simulink model "sim_test"  (R2021a)
settings: Solver=VariableStepAuto  StartTime=0.0  StopTime=240  RelTol=1e-3
libraries: dspvision x1
settings Model: SimulationMode=accelerator  Creator=Rafid  LastModifiedBy=Rafid

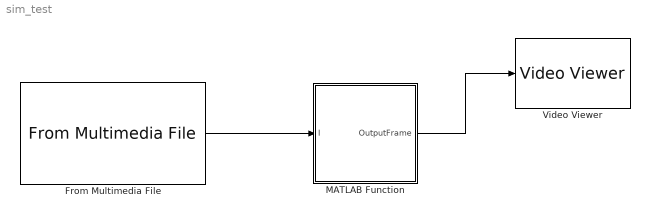
== system sim_test ==
  From Multimedia File : dspvision/From Multimedia File  inputFilename=C:\Users\Rafid\Documents\capstone\DroneCapture2.mp4  readRange=[1 Inf]  loop=on  numPlays=inf  outputStreams=Video only  videoDataType=single  audioDataType=int16  inheritSampleTime=on  userDefinedSampleTime=1/30  noAudioOutput=off  isIntensityVideo=off  fourcc=RGB  colorVideoFormat=One multidimensional signal  outputEOF=off  dataOrg=Column-major  audioFrameSize=1024  computeAudioFrameSize=off  outSamplingMode=Sample based
  MATLAB Function : MATLAB Function  TreatAsAtomicUnit=on
  Video Viewer : VideoViewer  FigPos=[-1919 1461.33333333333 1920 952.666666666667]
  wires:
  MATLAB Function/1(OutputFrame) -> Video Viewer/1
  From Multimedia File/1 -> MATLAB Function/1(I)

== matlab function sim_test/MATLAB Function ==
  data: I input; OutputFrame output
function OutputFrame = fcn(I)
    OutputFrame = ones(size(I));
    coder.extrinsic('get_object');
    tic
    OutputFrame = get_object(I);
    toc
end
